simulink model "robosim"  (R2024b)
settings: Solver=VariableStepAuto  StartTime=0.0  StopTime=inf  RelTol=1e-3
libraries: vrlib x1
settings Model: Creator=HUAWEI  LastModifiedBy=HUAWEI

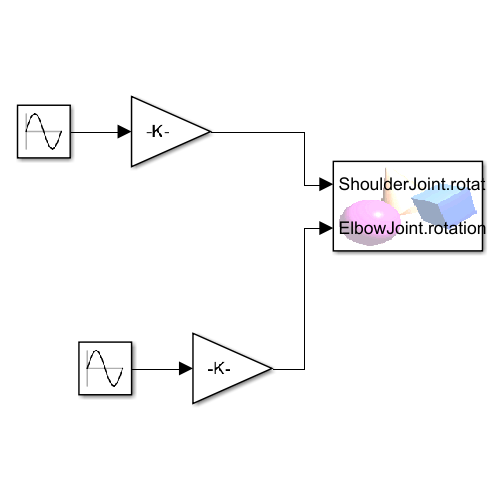
[thumbnail: Simulink's stored preview of the top-level diagram]
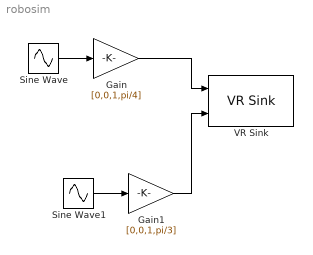
== system robosim ==
  Gain : Gain  Gain=[0,0,1,pi/4]
  Gain1 : Gain  Gain=[0,0,1,pi/3]
  Sine Wave : Sin  Frequency=0.1*2*pi  Phase=1  SampleTime=0
  Sine Wave1 : Sin  Frequency=0.1*2*pi  Phase=1  SampleTime=0
  VR Sink : vrlib/VR Sink  InstantiateOnLoad=on  SampleTime=0.1  ViewEnable=on  RemoteChange=off  RemoteView=off  FieldsWritten=ShoulderJoint.rotation.4.1.1.double#ElbowJoint.rotation.4.1.1.double  WorldFileName=w13_m1_SCARA.x3d  AutoView=off  VideoDimensions=[]  AllowVariableSize=off
  wires:
  Gain/1 -> VR Sink/1
  Gain1/1 -> VR Sink/2
  Sine Wave/1 -> Gain/1
  Sine Wave1/1 -> Gain1/1
